simulink model "HeartModel"  (R2014a)
settings: Solver=FixedStepDiscrete  StartTime=0.0  StopTime=100  FixedStep=0.01  RelTol=1e-3
settings Model: Creator=alexandru  LastModifiedBy=alexandru
settings DataIOCC: LimitDataPoints=off  SaveOutput=off  SignalLogging=off  DSMLogging=off  SaveTime=off
settings HardwareCC: TargetBitPerLong=64  TargetBitPerPointer=64  TargetLongLongMode=on  TargetIntDivRoundTo=Zero  TargetEndianess=LittleEndian  TargetWordSize=64  TargetHWDeviceType=MATLAB Host  ProdEqTarget=off
settings RTWCC: SystemTargetFile=rsim.tlc  GenCodeOnly=on  PackageGeneratedCodeAndArtifacts=on  PackageName=idhp_model_heart_realtime  TemplateMakefile=rsim_default_tmf  Description=Rapid Simulation Target  ProcessScript=rsim_make_rtw_hook
settings RSimTargetCC: ERTMultiwordTypeDef=System defined  ERTMultiwordLength=256  EnableShiftOperators=on

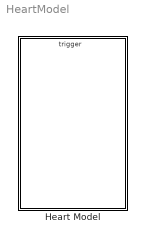
== system HeartModel ==
  Heart Model : Stateflow chart  Priority=1  TreatAsAtomicUnit=on

== stateflow chart HeartModel/Heart Model ==
  state Heart
    state A_dV [parallel]
      settings: executionOrder=13
      state a_dVLow
      state a_dvHigh
      (default) -> a_dVLow
      a_dVLow -> a_dvHigh [order 1] : a_dVSetHigh
      a_dVLow -> a_dVLow [order 2] : tr_AVJ
          | {send(AVJAnteReached,AVJ);}
      a_dvHigh -> a_dvHigh [order 2] : tr_AVJ
          | {send(AVJAnteReachedHigh,AVJ);}
      a_dvHigh -> a_dVLow [order 1] : a_dVSetLow
    state VtrNoiseGenerator [parallel]
      settings: executionOrder=3
      state q0
      (default) -> Heart.VtrNoiseGenerator.q0
      Heart.VtrNoiseGenerator.q0 -> Heart.VtrNoiseGenerator.q0 : after(VRG_noiseD, msec)
    state VRGEctopic [parallel]
      settings: executionOrder=10
      state q0
      (default) -> Heart.VRGEctopic.q0
      Heart.VRGEctopic.q0 -> Heart.VRGEctopic.q0 : after(VRG_ectopD, msec)
          | {send(Vbeat,Ventricle);}
    state RAConductor [parallel]
      settings: executionOrder=6
      state Empty
      state Ante
      state Retro
      (default) -> Heart.RAConductor.Empty
      Heart.RAConductor.Empty -> Heart.RAConductor.Ante [order 1] : arg
      Heart.RAConductor.Ante -> Heart.RAConductor.Empty [order 1] : retroAVJ
      Heart.RAConductor.Empty -> Heart.RAConductor.Retro [order 2] : retroAVJ
      Heart.RAConductor.Retro -> Heart.RAConductor.Empty [order 1] : arg
      Heart.RAConductor.Retro -> Heart.RAConductor.Empty [order 2] : after(RA_retroD,msec)
          | {send(AtrRetroReached,...
          | Atrium);}
      Heart.RAConductor.Ante -> Heart.RAConductor.Empty [order 2] : after(RA_anteD,msec)
          | {send(tr_AVJ,A_dV);}
    state AVJOut [parallel]
      settings: executionOrder=4
      state Empty
      state Ante
      state Retro
      (default) -> Heart.AVJOut.Empty
      Heart.AVJOut.Ante -> Heart.AVJOut.Empty : after(AVJDelay(avj_tRec,...
          | AV_anteDMin),msec)
          | {send(anteAVJ,RVConductor);}
      Heart.AVJOut.Empty -> Heart.AVJOut.Ante [order 1] : AVJAnteExit
      Heart.AVJOut.Retro -> Heart.AVJOut.Empty : after(AVJDelay(avj_tRec,...
          | AV_retroDMin),msec)
          | {send(retroAVJ,...
          | RAConductor);}
      Heart.AVJOut.Empty -> Heart.AVJOut.Retro [order 2] : AVJRetroExit
    state RVConductor [parallel]
      settings: executionOrder=5
      state Empty
      state Ante
      state Retro
      (default) -> Heart.RVConductor.Empty
      Heart.RVConductor.Empty -> Heart.RVConductor.Ante [order 1] : anteAVJ
      Heart.RVConductor.Empty -> Heart.RVConductor.Retro [order 2] : vrg
      Heart.RVConductor.Ante -> Heart.RVConductor.Empty [order 1] : vrg
      Heart.RVConductor.Ante -> Heart.RVConductor.Empty [order 2] : after(RV_anteD,msec)
          | {send(VtrAnteReached,...
          | Ventricle);}
      Heart.RVConductor.Retro -> Heart.RVConductor.Empty [order 1] : anteAVJ
      Heart.RVConductor.Retro -> Heart.RVConductor.Empty [order 2] : after(RV_retroD,msec)
          | {send(AVJRetroReached,...
          | AVJ);}
    state SANodeEctopic [parallel]
      settings: executionOrder=2
      state q0
      (default) -> Heart.SANodeEctopic.q0
      Heart.SANodeEctopic.q0 -> Heart.SANodeEctopic.q0 : after(SA_ectopD, msec)
          | {send(Abeat,Atrium);
          | send(a_dVSetHigh,A_dV);}
    state AtrNoiseGenerator [parallel]
      settings: executionOrder=1
      state q0
      Heart.AtrNoiseGenerator.q0 -> Heart.AtrNoiseGenerator.q0 : after(SA_noiseD, msec)
      (default) -> Heart.AtrNoiseGenerator.q0
    state VRG [parallel]
      settings: executionOrder=11
      state Wait4VBeat
      state Wait4VSynch
      (default) -> Wait4VBeat
      Wait4VBeat -> Wait4VSynch [order 2] : after(VRG_d, msec)
          | {send(Vbeat,Ventricle);}
      Wait4VSynch -> Wait4VBeat : NextVtrBeat
      Wait4VBeat -> Wait4VBeat [order 1] : NextVtrBeat
    state SANode [parallel]
      settings: executionOrder=7
      state Wait4ABeat
      state Wait4ASynch
      (default) -> Wait4ABeat
      Wait4ABeat -> Wait4ASynch [order 2] : after(SA_d, msec)
          | {send(Abeat,Atrium);
          | send(a_dVSetLow,A_dV);
          | }
      Wait4ABeat -> Wait4ABeat [order 1] : NextAtrBeat
      Wait4ASynch -> Wait4ABeat : NextAtrBeat
    state AVJ [parallel]
      settings: executionOrder=12
      state Recovery
      state Ante
      state Refractory
      state Retro
      Heart.AVJ.Ante -> Heart.AVJ.Refractory : after(avj_t4,msec)
          | {ctime=ctime+temporalCount(msec);
          | avj_tRec=(ctime-recoverylast);
          | send(AVJAnteExit,AVJOut);
          | avj_refr_0=initRefrPeriod(avj_tRec);
          | avj_refr=avj_refr_0;
          | refractorylast=ctime;}
      Recovery -> Heart.AVJ.Ante [order 1] : AVJAnteReached{
          | ctime=ctime+temporalCount(msec);
          | avj_t4 = timeToDep(AV_Vr+ ...
          | (ctime-recoverylast)*AV_k4 + SA_dV);
          | }
      Recovery -> Heart.AVJ.Ante [order 3] : AVJAnteReachedHigh{
          | ctime=ctime+temporalCount(msec);
          | avj_t4 = timeToDep(AV_Vr+...
          | (ctime-recoverylast)*AV_k4 + SA_ectopdV);
          | }
      Heart.AVJ.Refractory -> Recovery [order 4] : after(avj_refr,msec){
          | ctime=ctime+temporalCount(msec);
          | avj_t4=timeToDep(AV_Vr);
          | recoverylast=ctime;
          | }
      (default) -> Recovery : {
          | avj_t4=timeToDep(AV_Vr);
          | ctime=0;
          | recoverylast=0;
          | refractorylast=0;
          | }
      Recovery -> Heart.AVJ.Retro [order 4] : AVJRetroReached{
          | ctime=ctime+temporalCount(msec);}
      Recovery -> Heart.AVJ.Refractory [order 2] : after(avj_t4,msec){
          | ctime=ctime+temporalCount(msec);
          | avj_tRec=avj_t4;
          | avj_refr_0=initRefrPeriod(avj_tRec);
          | avj_refr=avj_refr_0;
          | refractorylast=ctime;}
      Heart.AVJ.Refractory -> Heart.AVJ.Refractory [order 3] : AVJAnteReachedHigh
          | {ctime=ctime+temporalCount(msec);
          | avj_refr=avj_refr-(ctime - refractorylast)+...
          | modulateRefrAnte((ctime - refractorylast),...
          | avj_refr_0,SA_ectopdV);
          | refractorylast=ctime;
          | }
      Heart.AVJ.Refractory -> Heart.AVJ.Refractory [order 1] : AVJAnteReached
          | {ctime=ctime+temporalCount(msec);
          | avj_refr=avj_refr-(ctime - refractorylast)+...
          | modulateRefrAnte((ctime - refractorylast),...
          | avj_refr_0,SA_dV);
          | refractorylast=ctime;}
      Heart.AVJ.Refractory -> Heart.AVJ.Refractory [order 2] : AVJRetroReached
          | {ctime=ctime+temporalCount(msec);
          | avj_refr=avj_refr-(ctime - refractorylast)+...
          | modulateRefrRetro((ctime - refractorylast),...
          | avj_refr_0);
          | refractorylast=ctime;}
      Heart.AVJ.Retro -> Heart.AVJ.Refractory : {send(AVJRetroExit,AVJOut);
          | ctime=ctime+temporalCount(msec);
          | avj_tRec=ctime-recoverylast;
          | avj_refr_0=initRefrPeriod(avj_tRec);
          | avj_refr=avj_refr_0;
          | refractorylast=ctime;
          | }
    state Ventricle [parallel]
      settings: executionOrder=8
      state Excitable
      state Refractory
      state VsenseAnte
      state VSynch
      state Vsense
      state GenerateRetroWave
      (default) -> Heart.Ventricle.Refractory
      Heart.Ventricle.Refractory -> Heart.Ventricle.Excitable : after(Vtr_refrD,msec)
      Heart.Ventricle.Excitable -> GenerateRetroWave [order 2] : VP
      Heart.Ventricle.Excitable -> Vsense [order 3] : Vbeat
      Heart.Ventricle.Excitable -> VsenseAnte [order 1] : VtrAnteReached
      VSynch -> Heart.Ventricle.Refractory : {send(NextVtrBeat,...
          | VRG);}
      VsenseAnte -> VSynch : {SWrite(0x32);}
      GenerateRetroWave -> VSynch : {send(vrg,RVConductor);}
      Vsense -> GenerateRetroWave : {SWrite( 0x32);}
    state Atrium [parallel]
      settings: executionOrder=9
      state Excitable
      state Refractory
      state AsenseRetro
      state ASynch
      state Asense
      state GenerateAnteWave
      (default) -> Heart.Atrium.Refractory
      Heart.Atrium.Excitable -> Asense [order 1] : Abeat
      Heart.Atrium.Refractory -> Heart.Atrium.Excitable : after(Atr_refrD,msec)
      Heart.Atrium.Excitable -> AsenseRetro [order 3] : AtrRetroReached
      ASynch -> Heart.Atrium.Refractory : {send(NextAtrBeat,...
          | SANode);}
      Heart.Atrium.Excitable -> GenerateAnteWave [order 2] : AP
      AsenseRetro -> ASynch : {SWrite(0x31);}
      GenerateAnteWave -> ASynch : {send(arg,RAConductor);}
      Asense -> GenerateAnteWave : {SWrite(0x31);}
    state Parameter_Serial [parallel]
      settings: executionOrder=14
      state Init
      state DataReceived
      DataReceived -> Init [order 3] : [bufs1==0x34]
          | {send(VP, Ventricle);}
      Init -> DataReceived : SREC
          | {bufs1 = SReceive();}
      (default) -> Init
      DataReceived -> Init [order 2] : [bufs1==0x33]
          | {send(AP, Atrium);}
      DataReceived -> Init [order 1] : [(bufs1!=0x33 && bufs1!=0x34)]
  (default) -> Heart
  data: t function_output double; tRec function_input double; minDly function_input double; t function_output double; Vm function_input double; t function_input double; t0 function_input double; dT function_output double; dV function_input double; t function_input double; dT function_output double; t0 function_input double; t function_output double; tRec function_input double; stat function_output double; c function_input double; value function_input double; stat function_output double; h function_input double; buf function_output double; stat function_output double; h function_input double; d function_input double; e function_input double; Atr_refrD local double =50; AV_alpha local double =150; AV_anteDMin local double =50; AV_beta local double =250; AV_delta local double =10; AV_k4 local double =0.03; AV_refrDMin local double =50; AV_retroDMin local double =100; AV_tauC local double =100; AV_theta local double =10; AV_tr local double =500; AV_Vr local double =-90; AV_Vt local double =-40; RA_anteD local double =30; RA_retroD local double =30; RV_anteD local double =50; RV_retroD local double =50; SA_d local double =1000; SA_dV local double =50; SA_ectopD local double =10400; SA_ectopdV local double =50; SA_noiseD local double =1000000; VRG_d local double =3000; VRG_ectopD local double =30450; VRG_noiseD local double =1000000; Vtr_refrD local double =200; avj_tRec local double; clk local double; recoverylast local double; avj_t4 local double; ctime local double; avj_refr local double; avj_refr_0 local double; refractorylast local double; BAUDRATE local uint32 =57600; bufs1 local uint8; bufs2 local uint8; bufs3 local uint8; bufs4 local uint8; bufs5 local uint8; parid local uint16; value local uint32; parval local double; tmp16 local uint16; tmp32 local uint32
  events: Abeat local FUNCTION_CALL_EVENT; AtrRetroReached local FUNCTION_CALL_EVENT; arg local FUNCTION_CALL_EVENT; retroAVJ local FUNCTION_CALL_EVENT; AVJAnteReached local FUNCTION_CALL_EVENT; NextAtrBeat local FUNCTION_CALL_EVENT; AVJRetroReached local FUNCTION_CALL_EVENT; anteAVJ local FUNCTION_CALL_EVENT; vrg local FUNCTION_CALL_EVENT; VtrAnteReached local FUNCTION_CALL_EVENT; AVJRetroExit local FUNCTION_CALL_EVENT; AVJAnteExit local FUNCTION_CALL_EVENT; NextVtrBeat local FUNCTION_CALL_EVENT; Vbeat local FUNCTION_CALL_EVENT; AP local EITHER_EDGE_EVENT; VP local EITHER_EDGE_EVENT; AS local RISING_EDGE_EVENT; VS local RISING_EDGE_EVENT; Aget local EITHER_EDGE_EVENT; Vget local EITHER_EDGE_EVENT; Aintrinsic local EITHER_EDGE_EVENT; Anoise local EITHER_EDGE_EVENT; Aretro local EITHER_EDGE_EVENT; Vintrinsic local EITHER_EDGE_EVENT; Vnoise local EITHER_EDGE_EVENT; APElectr local RISING_EDGE_EVENT; VPElectr local EITHER_EDGE_EVENT; IncrClk local FUNCTION_CALL_EVENT; State local FUNCTION_CALL_EVENT; Clk0 local FUNCTION_CALL_EVENT; Clk1 local FUNCTION_CALL_EVENT; a_dVSetHigh local FUNCTION_CALL_EVENT; a_dVSetLow local FUNCTION_CALL_EVENT; tr_AVJ local FUNCTION_CALL_EVENT; AVJAnteReachedHigh local FUNCTION_CALL_EVENT; RLRI local FUNCTION_CALL_EVENT; TAVI local FUNCTION_CALL_EVENT; RTAVI local FUNCTION_CALL_EVENT; RURI local FUNCTION_CALL_EVENT; SREC input FUNCTION_CALL_EVENT
  function t  = AVJDelay(tRec,minDly):
    | function t  = AVJDelay(tRec,minDly)
    |     t = minDly+AV_alpha*exp(-tRec/AV_tauC);
    | end
  function t  = timeToDep(Vm):
    | function t  = timeToDep(Vm)
    |     t = max(0,(AV_Vt-Vm)/AV_k4);
    | end
  function dT  = modulateRefrAnte(t,t0,dV):
    | function dT  = modulateRefrAnte(t,t0,dV)
    |     %val1 = t/t0;
    |     %val2 = power(t/t0,avj_theta);
    |     dT = AV_refrDMin*power(t/t0,AV_theta)*power(min(1,dV/(AV_Vt-AV_Vr)),AV_delta);
    |     %fprintf(1,'%f %f\n', val1, val2);
    | end
  function dT  = modulateRefrRetro(t,t0):
    | 
    | function dT  = modulateRefrRetro(t,t0)
    |     dT = AV_refrDMin*power(t/t0,AV_theta);
    | end
  function t  = initRefrPeriod(tRec):
    | function t  = initRefrPeriod(tRec)
    |     t = AV_refrDMin + AV_beta*(1 - exp(-tRec/AV_tr));
    | end
  function stat  = SetParameters(c, value):
    | function stat  = SetParameters(c, value)
    | stat  = 0;
    | end
  function stat  = SWrite(h):
    | function stat  = SWrite(h)
    | stat = 0;
    | end
  function buf  = SReceive:
    | function buf  = SReceive()
    |     buf = 0;
    | end
  function stat  = SWrite3(h,d,e):
    | function stat  = SWrite3(h,d,e)
    | stat = 0;
    | end
